simulink model "ForErik_14b"  (R2014b)
settings: Solver=ode3  SolverMode=SingleTasking  StartTime=0.0  StopTime=100.0  FixedStep=0.001  RelTol=1e-3
values from neighbouring files (symbols this model uses):
  A_disk = kest.a    [TestKalman.m]
  b = 0.1    [Input_LQR.m]    (also in TestKalman.m; TestSuper.m; TestVahidComparison.m; parameter.m)
  B_disk = kest.b    [TestKalman.m]
  C_disk = C_disk(1:2,:)    [TestKalman.m]
  delta = cell(1,length(L_sup))    [TestSuper.m]
  g = 9.81    [Input_LQR.m]    (also in TestKalman.m; TestSuper.m; TestVahidComparison.m; parameter.m = 9.8)
  gamma = cell(1,length(L_sup))    [TestSuper.m]
  h = 0.01    [Input_LQR.m]    (also in TestKalman.m = 0.001; TestSuper.m = 0.001; TestVahidComparison.m = 0.001; parameter.m)
  H = [1 0 0 0 0 0 ... (first row only)    [Input_LQR.m]    (also in TestKalman.m; TestSuper.m; TestVahidComparison.m)
  k = 0.15    [Input_LQR.m]    (also in TestKalman.m; TestSuper.m; TestVahidComparison.m; parameter.m)
  m = 3/4    (= 0.75)    [Input_LQR.m]    (also in TestKalman.m; TestSuper.m; TestVahidComparison.m; parameter.m)
  M = 1    [Input_LQR.m]    (also in TestKalman.m; TestSuper.m; TestVahidComparison.m; parameter.m)
  P_0 = diag([1,1,1,1,1,1])*0.00001    [Input_LQR.m]    (also in TestKalman.m = diag([1,1,1,1,100,100])*0.001; TestSuper.m = diag([1,1,1,1,100,100])*0.001)
  phi = cell(1,length(L_sup))    [TestSuper.m]
  Q_kalman = diag([(0), (0)])    [Input_LQR.m]    (also in TestKalman.m = diag([(10), (10e-4)]); TestSuper.m = diag([(10), (10e-4)]))
  R_kalman = diag([(10e-7), (10e-6)])    [Input_LQR.m]    (also in TestKalman.m = diag([(10e-7), (10e-7)]); TestSuper.m = diag([(10e-7), (10e-7)]))
  X_0 = [0 0 0 0 0 0]'    [Input_LQR.m]    (also in TestKalman.m = [x_0 theta_0 x_dot0 theta_dot0 0 0]'; TestSuper.m = [x_0 theta_0 x_dot0 theta_dot0 0 0]')
  y_0 = [0 0]    [Input_LQR.m]    (also in TestKalman.m; TestSuper.m)
undefined symbols (not defined in the file or in its folder): A_kA2, A_ss, B_kA2, B_ss, C_kA2, C_ss, D_kA2, D_ss, L_kalman
libraries: simulink x4
settings Model: CovMetricSettings=dwe  CovHtmlReporting=off  covSaveCumulativeToWorkspaceVar=off  CovSaveSingleToWorkspaceVar=off  CovExternalEMLEnable=on  CovSFcnEnable=on  Creator=vahhas  LastModifiedBy=Erik
settings DataIOCC: LimitDataPoints=off  SaveFormat=StructureWithTime
settings DebuggingCC: SolverPrmCheckMsg=none  FrameProcessingCompatibilityMsg=error  SFUnexpectedBacktrackingDiag=error  SFNoUnconditionalDefaultTransitionDiag=error
settings HardwareCC: ProdBitPerPointer=64  ProdLargestAtomicFloat=Float  ProdIntDivRoundTo=Zero  ProdEndianess=LittleEndian  ProdHWDeviceType=Specified
settings ModelReferenceCC: PropagateSignalLabelsOutOfModel=on
settings GRTTargetCC: TargetLangStandard=C99 (ISO)  GeneratePreprocessorConditionals=Use local settings

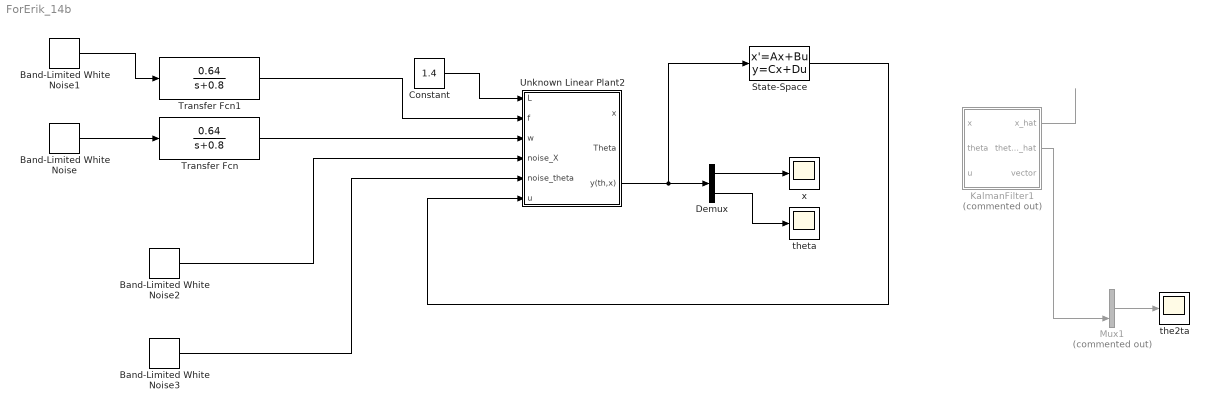
== system ForErik_14b ==
  Band-Limited White Noise : simulink/Sources/Band-Limited White Noise  Cov=10e-4  Ts=h  seed=[23343]
  Band-Limited White Noise1 : simulink/Sources/Band-Limited White Noise  Cov=10  Ts=h  seed=[23344]
  Band-Limited White Noise2 : simulink/Sources/Band-Limited White Noise  Cov=10e-7  Ts=h  seed=[23343]
  Band-Limited White Noise3 : simulink/Sources/Band-Limited White Noise  Cov=10e-7  Ts=h  seed=[23344]
  Constant : Constant  Value=1.4
  Demux : Demux  Outputs=2
  KalmanFilter1 : Subsystem  Commented=on
  Mux1 : Mux  Commented=on  Inputs=2
  State-Space : StateSpace  A=A_kA2  B=B_kA2  C=C_kA2  D=D_kA2  X0=0
  Transfer Fcn : TransferFcn  Numerator=[0.64]  Denominator=[1 0.8]
  Transfer Fcn1 : TransferFcn  Numerator=[0.64]  Denominator=[1 0.8]
  Unknown Linear Plant2 : Subsystem
  the2ta : Scope
  theta : Scope
      settings: SaveName=ScopeData2
  x : Scope
  wires:
  Unknown Linear Plant2/3(y(th,x)) -> Demux/1, State-Space/1
  State-Space/1 -> Unknown Linear Plant2/6(u)
  Band-Limited White Noise/1 -> Transfer Fcn/1
  Band-Limited White Noise1/1 -> Transfer Fcn1/1
  Transfer Fcn1/1 -> Unknown Linear Plant2/2(f)
  Transfer Fcn/1 -> Unknown Linear Plant2/3(w)
  Constant/1 -> Unknown Linear Plant2/1(L)
  KalmanFilter1/1(x_hat) -> ?
  KalmanFilter1/2(theta_hat) -> Mux1/2
  Mux1/1 -> the2ta/1
  Band-Limited White Noise2/1 -> Unknown Linear Plant2/4(noise_X)
  Band-Limited White Noise3/1 -> Unknown Linear Plant2/5(noise_theta)
  Demux/1 -> x/1
  Demux/2 -> theta/1

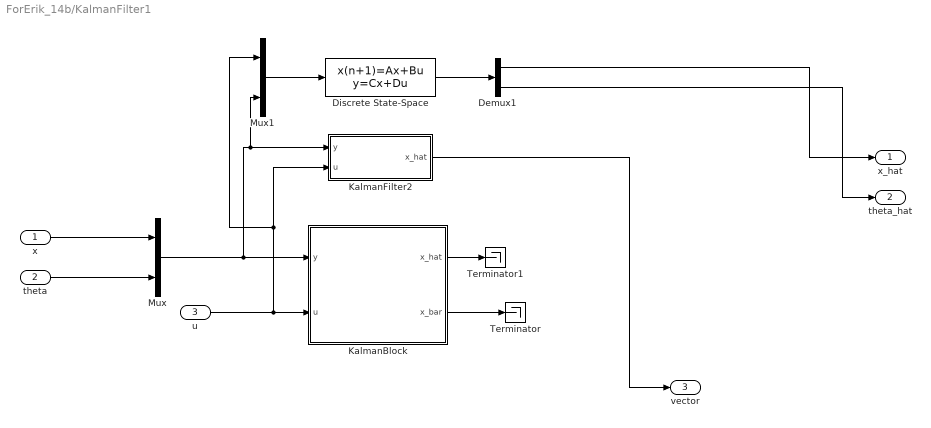
== system ForErik_14b/KalmanFilter1 ==
  x : Inport
  theta : Inport  Port=2
  "u " : Inport  Port=3
  Demux1 : Demux  Outputs=2
  Discrete State-Space : DiscreteStateSpace  A=A_ss  B=B_ss  C=C_ss  D=D_ss
  KalmanBlock : Subsystem
  KalmanFilter2 : Subsystem
  Mux : Mux  Inputs=2
  Mux1 : Mux  Inputs=2
  Terminator : Terminator
  Terminator1 : Terminator
  x_hat : Outport
  theta_hat : Outport  Port=2
  vector : Outport  Port=3
  wires:
  Mux/1 -> Mux1/2, KalmanFilter2/1(y), KalmanBlock/1("y ")
  x/1 -> Mux/1
  theta/1 -> Mux/2
  KalmanFilter2/1(x_hat) -> vector/1
  KalmanBlock/2(x_bar) -> Terminator/1
  KalmanBlock/1(x_hat) -> Terminator1/1
  Mux1/1 -> Discrete State-Space/1
  "u "/1 -> Mux1/1, KalmanFilter2/2(u), KalmanBlock/2("u ")
  Discrete State-Space/1 -> Demux1/1
  Demux1/1 -> x_hat/1
  Demux1/2 -> theta_hat/1

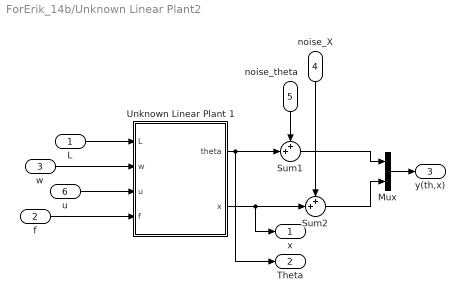
== system ForErik_14b/Unknown Linear Plant2 ==
  L : Inport
  f : Inport  Port=2
  w : Inport  Port=3
  noise_X : Inport  Port=4
  noise_theta : Inport  Port=5
  u : Inport  Port=6
  Mux : Mux  Inputs=2
  Sum1 : Sum  Inputs=++|
  Sum2 : Sum  Inputs=++|
  Unknown Linear Plant 1 : Subsystem
  x : Outport
  Theta : Outport  Port=2
  y(th,x) : Outport  Port=3
  wires:
  Mux/1 -> y(th,x)/1
  Sum2/1 -> Mux/2
  Sum1/1 -> Mux/1
  noise_X/1 -> Sum2/1
  Unknown Linear Plant 1/2(x) -> x/1, Sum2/2
  noise_theta/1 -> Sum1/1
  Unknown Linear Plant 1/1(theta) -> Theta/1, Sum1/2
  w/1 -> Unknown Linear Plant 1/2(w)
  L/1 -> Unknown Linear Plant 1/1(L)
  u/1 -> Unknown Linear Plant 1/3(u)
  f/1 -> Unknown Linear Plant 1/4(f)

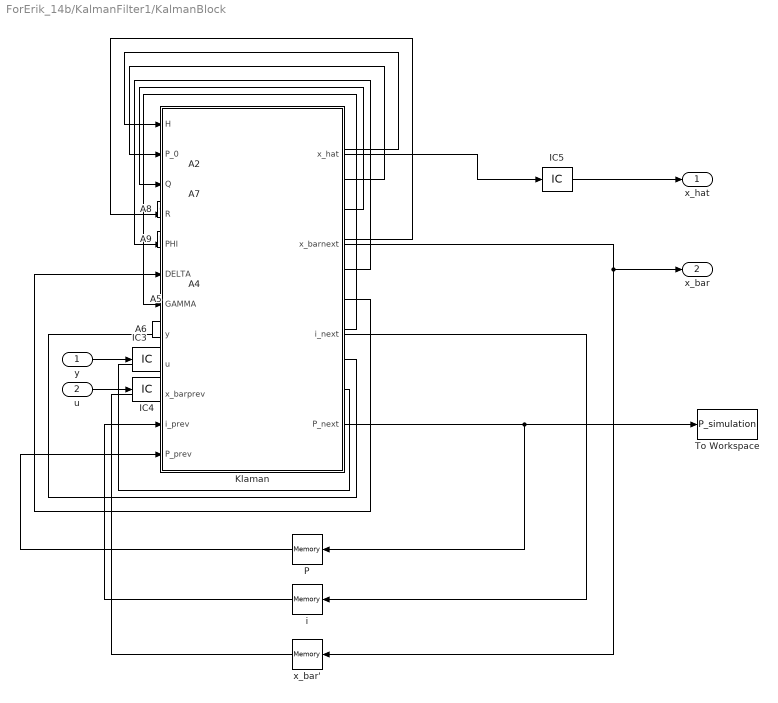
== system ForErik_14b/KalmanFilter1/KalmanBlock ==
  "y " : Inport
  "u " : Inport  Port=2
  A2 : Constant  Value=H
  A4 : Constant  Value=phi
  A5 : Constant  Value=delta
  A6 : Constant  Value=gamma
  A7 : Constant  Value=P_0
  A8 : Constant  Value=Q_kalman
  A9 : Constant  Value=R_kalman
  IC3 : InitialCondition  Value=y_0
  IC4 : InitialCondition  Value=0
  IC5 : InitialCondition  Value=X_0
  Klaman : MATLAB Function  TreatAsAtomicUnit=on
  P : Memory  X0=P_0
  To Workspace : ToWorkspace  VariableName=P_simulation  SampleTime=-1
  "i " : Memory
  x_bar' : Memory  X0=X_0
  x_hat : Outport
  x_bar : Outport  Port=2
  wires:
  A8/1 -> Klaman/3(Q)
  A6/1 -> Klaman/7(GAMMA)
  A4/1 -> Klaman/5(PHI)
  Klaman/2(x_barnext) -> x_bar'/1, x_bar/1
  Klaman/3(i_next) -> "i "/1
  Klaman/1(x_hat) -> IC5/1
  A2/1 -> Klaman/1(H)
  A5/1 -> Klaman/6(DELTA)
  IC4/1 -> Klaman/9(u)
  A7/1 -> Klaman/2(P_0)
  "u "/1 -> IC4/1
  A9/1 -> Klaman/4(R)
  "y "/1 -> IC3/1
  IC5/1 -> x_hat/1
  IC3/1 -> Klaman/8(y)
  "i "/1 -> Klaman/11(i_prev)
  P/1 -> Klaman/12(P_prev)
  x_bar'/1 -> Klaman/10(x_barprev)
  Klaman/4(P_next) -> P/1, To Workspace/1

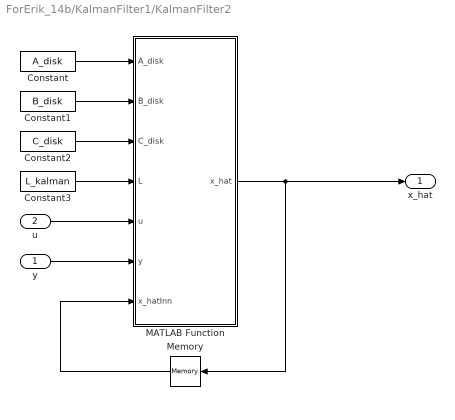
== system ForErik_14b/KalmanFilter1/KalmanFilter2 ==
  y : Inport
  u : Inport  Port=2
  Constant : Constant  Value=A_disk
  Constant1 : Constant  Value=B_disk
  Constant2 : Constant  Value=C_disk
  Constant3 : Constant  Value=L_kalman
  MATLAB Function : MATLAB Function  TreatAsAtomicUnit=on
  Memory : Memory  X0=X_0
  x_hat : Outport
  wires:
  Constant/1 -> MATLAB Function/1(A_disk)
  Constant1/1 -> MATLAB Function/2(B_disk)
  Constant2/1 -> MATLAB Function/3(C_disk)
  Constant3/1 -> MATLAB Function/4(L)
  MATLAB Function/1(x_hat) -> Memory/1, x_hat/1
  Memory/1 -> MATLAB Function/7(x_hatInn)
  u/1 -> MATLAB Function/5(u)
  y/1 -> MATLAB Function/6(y)

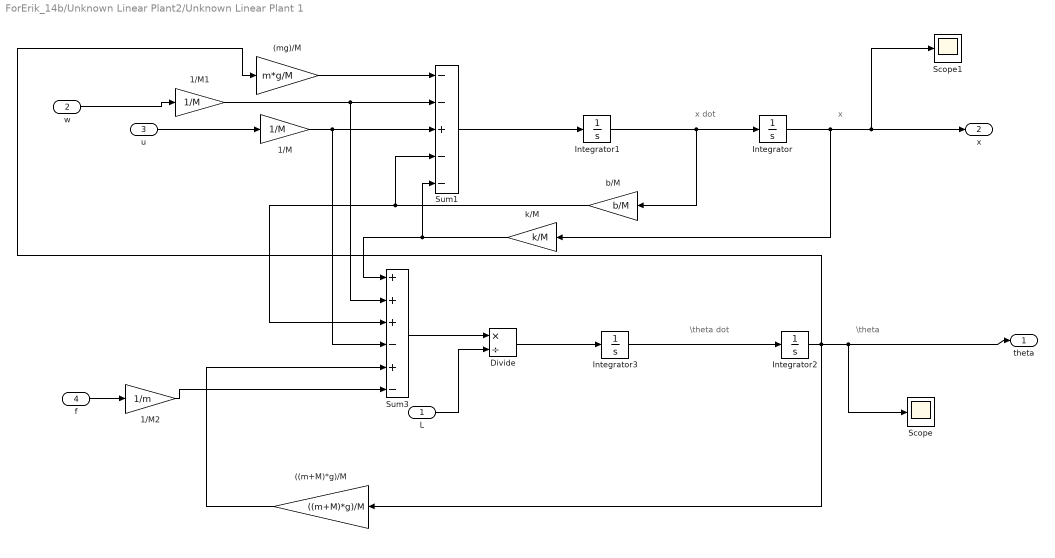
== system ForErik_14b/Unknown Linear Plant2/Unknown Linear Plant 1 ==
  note: \theta dot
  note: x dot
  note: \theta
  note: x
  L : Inport
  w : Inport  Port=2
  u : Inport  Port=3
  f : Inport  Port=4
  ((m+M)*g)/M : Gain  Gain=((m+M)*g)/M
  (mg)/M : Gain  Gain=m*g/M
  1/M : Gain  Gain=1/M
  1/M1 : Gain  Gain=1/M
  1/M2 : Gain  Gain=1/m
  Divide : Product  Inputs=*/
  Integrator{,1..3} (4 alike) : Integrator
  Scope : Scope
      settings: YMin=0  YMax=32.5  SaveName=ScopeData4
  Scope1 : Scope
      settings: YMin=0.12  YMax=0.175  SaveName=ScopeData5
  Sum1 : Sum  Inputs=--+--
  Sum3 : Sum  Inputs=+++-+-
  b/M : Gain  Gain=b/M
  k/M : Gain  Gain=k/M
  theta : Outport
  x : Outport  Port=2
  wires:
  k/M/1 -> Sum3/1, Sum1/5
  Integrator3/1 -> Integrator2/1
  Integrator1/1 -> Integrator/1, b/M/1
  Integrator/1 -> k/M/1, Scope1/1, x/1
  Integrator2/1 -> Scope/1, theta/1, (mg)/M/1, ((m+M)*g)/M/1
  u/1 -> 1/M/1
  b/M/1 -> Sum3/3, Sum1/4
  1/M/1 -> Sum3/4, Sum1/3
  w/1 -> 1/M1/1
  1/M1/1 -> Sum3/2, Sum1/2
  (mg)/M/1 -> Sum1/1
  Sum1/1 -> Integrator1/1
  Sum3/1 -> Divide/1
  Divide/1 -> Integrator3/1
  L/1 -> Divide/2
  ((m+M)*g)/M/1 -> Sum3/5
  f/1 -> 1/M2/1
  1/M2/1 -> Sum3/6

== matlab function ForErik_14b/KalmanFilter1/KalmanBlock/Klaman ==
  data: H input; P_0 input; Q input; R input; PHI input; DELTA input; GAMMA input; y input; u input; x_barprev input; i_prev input; P_prev input; x_hat output; x_barnext output; i_next output; P_next output
function [x_hat, x_barnext, i_next, P_next] = KalmanFilter(H, P_0, Q, R, PHI, DELTA, GAMMA, y, u, x_barprev, i_prev, P_prev)
I = eye(6);
if i_prev == 0
    x_barnext = x_barprev;
    x_hat = x_barprev;
    P_next = P_0;
else
    K = P_prev * (H') * inv(H * P_prev * (H') + R);
    x_hat = x_barprev + K * (y - H * x_barprev);
    P_hat = (I - K * H) * P_prev * (I - K * H)' + K * R * K';
        
    x_barnext = PHI * x_hat + DELTA * u;
    P_next = PHI * P_hat * PHI' + GAMMA * Q * GAMMA';
end

i_next=i_prev+1;
end

== matlab function ForErik_14b/KalmanFilter1/KalmanFilter2/MATLAB Function ==
  data: A_disk input; B_disk input; C_disk input; L input; u input; y input; x_hat output; x_hatInn input
function x_hat = fcn(A_disk,B_disk,C_disk,L,u,y,x_hatInn)

x_hat=A_disk*x_hatInn+B_disk(:,1)*u+L*(y-C_disk*x_hatInn);

end
